simulink model "example"  (Simulink 9.3)
settings: Solver=VariableStepAuto  StartTime=0.0  StopTime=10.0  RelTol=1e-3
settings Model: Creator=jhu  LastModifiedBy=msayers
settings DataIOCC: SaveFormat=Dataset  SignalLoggingSaveFormat=Dataset  ReturnWorkspaceOutputs=on
settings OptimizationCC: LifeSpan=auto
settings DebuggingCC: UnderspecifiedInitializationDetection=Simplified  MergeDetectMultiDrivingBlocksExec=error  FcnCallInpInsideContextMsg=error  UnconnectedInputMsg=none  UnconnectedOutputMsg=none  UnconnectedLineMsg=none  SFUnexpectedBacktrackingDiag=error  SFNoUnconditionalDefaultTransitionDiag=error  SFExecutionAtInitializationDiag=warning  SFMachineParentedDataDiag=error
settings HardwareCC: ProdBitPerPointer=64  ProdBitPerSizeT=64  ProdBitPerPtrDiffT=64  ProdLargestAtomicFloat=Float  ProdIntDivRoundTo=Zero  ProdEndianess=LittleEndian  ProdWordSize=64  ProdHWDeviceType=Intel->x86-64 (Windows64)
settings ModelReferenceCC: PropagateSignalLabelsOutOfModel=on
settings SFSimCC: SimUseLocalCustomCode=on
settings RTWCC: RTWUseLocalCustomCode=on
settings CodeAppCC: StateflowObjectComments=off
settings GRTTargetCC: TargetLangStandard=C99 (ISO)  CombineOutputUpdateFcns=on  GRTInterface=off
settings ConfigComp: CovMetricSettings=dwe  CovHtmlReporting=off  CovSaveCumulativeToWorkspaceVar=off  CovSaveSingleToWorkspaceVar=off  CovExternalEMLEnable=on

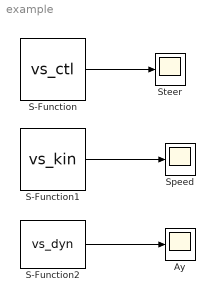
== system example ==
  Ay : Scope
  S-Function : S-Function  Priority=1  FunctionName=vs_ctl  Parameters='simfile.sim'  SFunctionDeploymentMode=off  EnableBusSupport=off
  S-Function1 : S-Function  Priority=2  FunctionName=vs_kin  Parameters='simfile.sim'  SFunctionDeploymentMode=off  EnableBusSupport=off
  S-Function2 : S-Function  Priority=3  FunctionName=vs_dyn  Parameters='simfile.sim'  SFunctionDeploymentMode=off  EnableBusSupport=off
  Speed : Scope
  Steer : Scope
  wires:
  S-Function/1 -> Steer/1
  S-Function2/1 -> Ay/1
  S-Function1/1 -> Speed/1
